simulink model "lateral_747"  (Simulink 7.8)
settings: Solver=ode45  StartTime=0.0  StopTime=10.0  RelTol=1e-3
undefined symbols (not defined in the file): Gwo_r, syslatr
settings Model: Creator=Dan  LastModifiedBy=Dan
settings DebuggingCC: InitInArrayFormatMsg=none

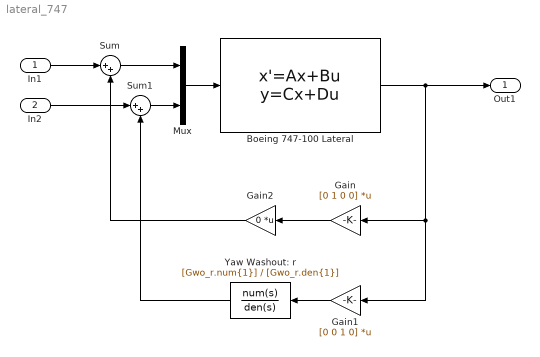
== system lateral_747 ==
  In1 : Inport
  In2 : Inport  Port=2
  "Boeing 747-100 Lateral " : StateSpace  A=syslatr.A  B=syslatr.B  C=syslatr.C  D=syslatr.D
  Gain : Gain  Gain=[0 1 0 0]  Multiplication=Matrix(K*u)
  Gain1 : Gain  Gain=[0 0 1 0]  Multiplication=Matrix(K*u)
  Gain2 : Gain  Gain=0  Multiplication=Matrix(K*u)
  Mux : Mux  Inputs=2
  Sum : Sum  Inputs=|++
  Sum1 : Sum  Inputs=|++
  Yaw Washout: r : TransferFcn  Numerator=[Gwo_r.num{1}]  Denominator=[Gwo_r.den{1}]
  Out1 : Outport
  wires:
  Sum/1 -> Mux/1
  Sum1/1 -> Mux/2
  "Boeing 747-100 Lateral "/1 -> Gain/1, Gain1/1, Out1/1
  Gain/1 -> Gain2/1
  Gain1/1 -> Yaw Washout: r/1
  In1/1 -> Sum/1
  In2/1 -> Sum1/1
  Gain2/1 -> Sum/2
  Yaw Washout: r/1 -> Sum1/2
  Mux/1 -> "Boeing 747-100 Lateral "/1
